simulink model "acc"  (R2024b)
settings: Solver=VariableStepAuto  StartTime=0.0  StopTime=80  RelTol=1e-3
libraries: SignalEditorBlockLib x3

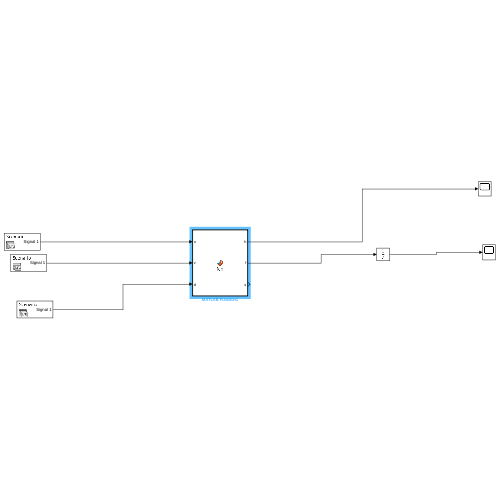
[thumbnail: Simulink's stored preview of the top-level diagram]
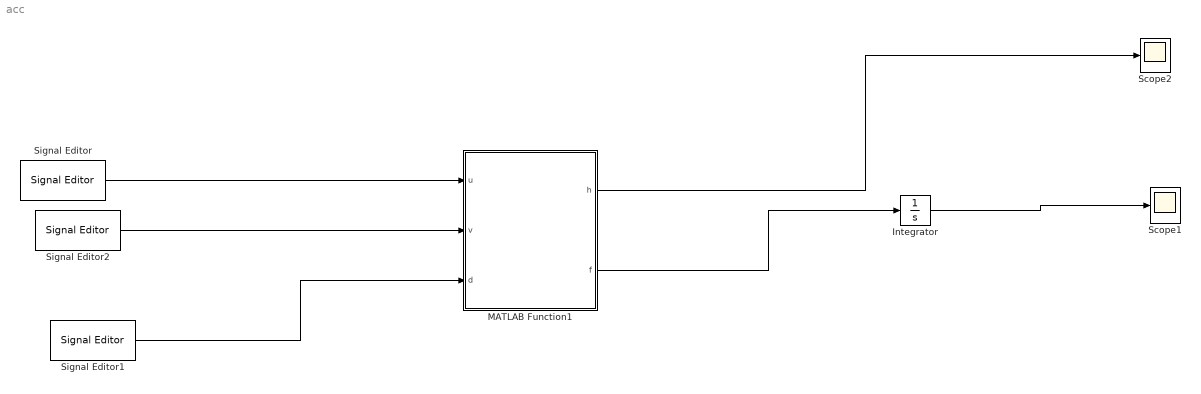
== system acc ==
  Integrator : Integrator
  MATLAB Function1 : MATLAB Function  TreatAsAtomicUnit=on
  Scope1 : Scope
  Scope2 : Scope
  Signal Editor : SignalEditorBlockLib/Signal Editor  FileName=signal1.mat  ActiveScenario=Scenario  ActiveSignal=Signal 1  IsBus=off  OutputBusObjectStr=Bus: BusObject  SampleTime=0  ZeroCross=off  OutputAfterFinalValue=Setting to zero  Unit=m/s  PreserveSignalName=on  ApplySigPropsToAllScenarios=on  ApplySigPropsToAllSignals=off
  Signal Editor1 : SignalEditorBlockLib/Signal Editor  FileName=signal2.mat  ActiveScenario=Scenario  ActiveSignal=Signal 1  IsBus=off  OutputBusObjectStr=Bus: BusObject  SampleTime=0  ZeroCross=off  OutputAfterFinalValue=Setting to zero  Unit=m  PreserveSignalName=on  ApplySigPropsToAllScenarios=on  ApplySigPropsToAllSignals=off
  Signal Editor2 : SignalEditorBlockLib/Signal Editor  FileName=signal3.mat  ActiveScenario=Scenario  ActiveSignal=Signal 1  IsBus=off  OutputBusObjectStr=Bus: BusObject  SampleTime=0  ZeroCross=off  OutputAfterFinalValue=Setting to zero  Unit=m/s  PreserveSignalName=on  ApplySigPropsToAllScenarios=on  ApplySigPropsToAllSignals=off
  wires:
  Signal Editor/1 -> MATLAB Function1/1(u)
  Integrator/1 -> Scope1/1
  MATLAB Function1/1(h) -> Scope2/1
  Signal Editor2/1 -> MATLAB Function1/2(v)
  MATLAB Function1/2(f) -> Integrator/1
  Signal Editor1/1 -> MATLAB Function1/3(d)

== matlab function acc/MATLAB Function1 ==
  data: u input; v input; h output; f output; d input
function [h, f] = fcn(u, v, d)

    s = d;
    Ve = u;
    Vl = v;
    Vcr = 27.77;
    delta = 2;
    a = 2;
    b = 2;

    T = 1.5;
    s0 = 2;

    B = Ve*T + (Ve*(Ve - Vl)) / (2 * sqrt(a * b));
    s1 = s0 + max(0, B);
    z = s1 / s;

    if Ve <= Vcr
        afree = a * (1 - (Ve / Vcr)^delta);
        if z >= 1
            derivative = a * (1 - z^2);
        else
            derivative = afree * (1 - z^(2 * a / afree));
        end
    else

        afree = (-b * (1 - (Vcr / Ve)^(a * delta / b)));

        if z >= 1
            derivative = afree + a * (1 - z^2);
        else
            derivative = afree;
        end
    end

    h = derivative;
  
    f = derivative;
    

end
